simulink library "Simple_lib"  (R2018b)
settings: Solver=ode45  StartTime=0.0  StopTime=10.0  RelTol=1e-3  EnableMultiTasking=on
undefined symbols (not defined in the file or in its folder): Acceptance, beta, C, C_J, C_P, c_wall, dGain, DiscIntNeverNeededParam, Duplex, Electrical_lib, grab, h_fe, i, i3, K_T, Kman, KmanCE, mu_s, n_rev, R_arm, Simplex, systemTs, tau_0, TinIC, Ts, w_0, wallMass, Watch_lib
libraries: $bdroot x407, PlantUtilityBlockset_lib x30, peGeneralControl x22, simulink x11
(part 2 of 14)

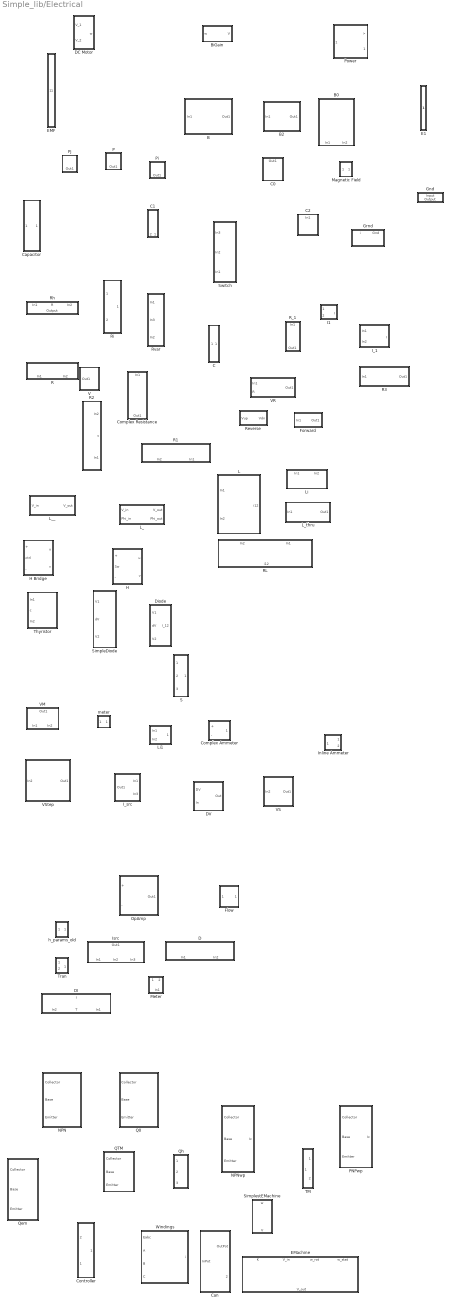
== system Simple_lib/Electrical ==
  B : Subsystem
      mask Display:
      | color('white')
      | plot([-1 1 1 -1 -1], [-1 -1 1 1 -1])
      | color('black')
      | 
      | plot([1.0 1.12 1.12 1.0], [0 .1 -.1 0])
      | plot([-1 -1], [-.4 .4])
      | plot([-.88 -.88], [-1 1])
      | plot([.88 .88], [-.4 .4])
      | plot([1 1], [-1 1])
      | 
      | plot([-.85 -.80], [0 0])
      | plot([-.7 -.6], [0 0])
      | plot([-.5 -.4], [0 0])
      | plot([-.3 -.2], [0 0])
      | plot([-.1 .0], [0 0])
      | plot([.1 .2], [0 0])
      | plot([.3 .4], [0 0])
      | plot([.5 .6], [0 0])
      | plot([.7 .8], [0 0])
  B0 : Subsystem
      mask Display:
      | color('white')
      | plot([-1 1 1 -1 -1], [-2 -2 2 2 -2])
      | color('black')
      | 
      | %plot( [0 .1 -.1 0],[1.0 1.12 1.12 1.0])
      | plot( [-.4 .4],[-.88 -.88])
      | plot([-1 1],[-1 -1])
      | plot([-.4 .4],[1 1])
      | plot([-1 1], [.88 .88])
      | 
      | plot([0 0],[-.85 -.80])
      | plot([0 0],[-.7 -.6])
      | plot([0 0],[-.5 -.4])
      | plot([0 0],[-.3 -.2])
      | plot([0 0],[-.1 .0])
      | plot([0 0],[.1 .2])
      | plot([0 0],[.3 .4])
      | plot([0 0],[.5 .6])
      | plot([0 0],[.7 .8])
  B2 : Subsystem
      mask Display:
      | plot([0 0], [-.4 .4])
      | plot([.06 .06], [-1 1])
      | plot([.94 .94], [-.4 .4])
      | 
      | plot([1 1], [-1 1])
      | plot([.06 .1], [0 0])
      | plot([.16 .2], [0 0])
      | plot([.26 .3], [0 0])
      | plot([.36 .4], [0 0])
      | plot([.46 .5], [0 0])
      | plot([.56 .6], [0 0])
      | plot([.66 .7], [0 0])
      | plot([.76 .8], [0 0])
      | plot([.86 .9], [0 0])
  BiGain : Subsystem  mask{k_level=-1, k_flow=-1}
      mask prompts: k_level "Potential Gain"; k_flow "Flow Gain"
      settings: AttributesFormatString="%<k_flow>   %<k_level>"
      mask Display:
      | patch( [0 1 0],[1 0 -1])
      | color('green')
      | plot( [0 -1 0],[1 0 -1])
  C : Subsystem  mask{C=100e-6}
      mask prompts: C "Capacitance"
      settings: AttributesFormatString=%<C>F
      mask Display:
      | %plot([1.0 1.8 1.8 1.0], [0 .1 -.1 0])
      | patch([-1 -1 -.7 -.7 -1], [-1 1 1 -1 -1])
      | patch([1 1 .7 .7 1], [-1 1 1 -1 -1])
  C0 : Subsystem
      mask Display:
      | plot(1-[0 0],[-1 1])
      | plot(1-[-0.4 -0.4],[-1 1])
      | plot(1-[0.6 0.6], [-0.6 0.6])
      | plot(1-[0.8 0.8],[-0.2 0.2])
      | 
      | plot(1-[-0.4 -1], [0 0])
      | plot(1-[0 0.6],[0 0])
  C1 : Subsystem  mask{C=1}
      mask prompts: C "Capacitance"
      mask Display:
      | color('white')
      | plot([-1 1 1 -1 -1], [-1 -1 1 1 -1])
      | color('black')
      | 
      | plot([-1 1], [0.5 0.5])
      | plot([-1 1], [-0.5 -0.5])
  C2 : Subsystem
      mask Display:
      | color('white')
      | plot([-1 1 1 -1 -1], [-1 -1 1 1 -1])
      | 
      | color('black')
      | %plot([1.0 1.18 1.18 1.0], [0 .15 -.15 0])
      | plot([0 0],[-1 1])
      | plot([-0.4 -0.4],[-1 1])
      | plot([0.6 0.6], [-0.6 0.6])
      | plot([0.8 0.8],[-0.2 0.2])
      | 
      | plot([-0.4 -1], [0 0])
      | plot([0 0.6],[0 0])
  Can : Subsystem  Tag=Electrical  AncestorBlock=Watch_lib/Acceptance  InitFcn=initCan
      mask Display:
      | %color('white')
      | %plot([0 3], [2 2])
      | %plot([0 3], [-2 -2])
      | %color('black')
      | 
      | plot([-1 -1 -.8 -.3 .3 .8 1 1], [1.5 -1.5 -1.8 -2 -2 -1.8 -1.5 1.5])
      | patch([-1 -.8 -.3 .3 .8 1 .8 .3 -.3 -.8 -1],[1.5 1.3 1.1 1.1 1.3 1.5 1.8 2 2 1.8 1.5])
  Capacitor : Subsystem  mask{C=.01}
      mask prompts: C "Capacitance"
      settings: AttributesFormatString=%<C>F
      mask Display:
      | %plot([1.0 1.8 1.8 1.0], [0 .1 -.1 0])
      | patch([-1 -1 -.7 -.7 -1], [-1 1 1 -1 -1])
      | patch([1 1 .7 .7 1], [-1 1 1 -1 -1])
  Complex Ammeter : Subsystem
      mask Display:
      | plot([-1 -.9 -.5 0 .5 .9 1  .9  .5  0 -.5 -.9 -1],      [ 0  .5 .9 1 .9 .5 0 -.5 -.9 -1 -.9 -.5  0]);
      | %plot([0 0], [0 -0.8])
      | %plot([0.2 0 -0.2], -[0.7 0.8 0.7])
      | port_label('input',1,'  +')
      | port_label('input',2,'  -')
      | disp('A')
  Complex Resistance : Subsystem  mask{R=0.01}
      mask prompts: R "Resistance"
      settings: AttributesFormatString=%<R> Ohm
      mask Display:
      | %color('black')
      | %plot([1.0 1.18 1.18 1.0], [0 .2 -.2 0])
      | plot([-8:8]/8, [0 1 0 -1 0 1 0 -1 0 1 0 -1 0 1 0 -1 0])
      | 
      | color('white')
      | plot([-1 1 1 -1 -1], [-1 -1 1 1 -1])
  Controller : Subsystem  InitFcn=initSimplex
      mask Display:
      | %color('white')
      | %plot([0 3], [2 2])
      | %plot([0 3], [-2 -2])
      | %color('black')
      | 
      | %plot([0 2 2 3], [1 1 0 0])
      | %plot([1 3 2 1 0 2], [0.6 0.6 0.4 0.6 0.4 0.4])
      | %patch([1 3 2],[0.6 0.6 0.4],[0,0,0])
      | %plot([0 1 1], [1 1 0.6])
      | %plot([1 1 0], [0.4 -1 -1])
      | 
      | plot( [0 0 0.15 .9 1 1 .9 0.15 0], [-.96 .96 1 .85 .8 -.8 -.85 -1 -.96])
      | patch( [.3 .4 .4 .3], [-.03 -.03 .03 .03])
      | patch( [.3 .4 .4 .3], [-.03 -.03 .03 .03]+.4)
      | patch( [.3 .4 .4 .3], [-.03 -.03 .03 .03]+.8)
      | patch( [.3 .4 .4 .3], [-.03 -.03 .03 .03]-.4)
      | patch( [.3 .4 .4 .3], [-.03 -.03 .03 .03]-.8)
      | patch( [.3 .4 .4 .3]+.4, [-.03 -.03 .03 .03]-.2)
      | patch( [.3 .4 .4 .3]+.4, [-.03 -.03 .03 .03]+.2)
      | patch( [.3 .4 .4 .3]+.4, [-.03 -.03 .03 .03]-.6)
      | patch( [.3 .4 .4 .3]+.4, [-.03 -.03 .03 .03]+.6)
  D : Subsystem
      mask Display:
      | plot( [ -1 0 0 ],[-1 -1 -0.3 ])
      | plot( [ 0 0 -1],[ 0.3 1 1])
      | plot( [ -1 1],-[1 1]*.3)
      | plot([-1 1 0 -1],[1 1 -1 1]*.3)
      | color('white')
      | plot([-1 1 1 -1 -1], [-1 -1 1 1 -1]*2)
      | %port_label('input', 1, '1')
  DC Motor : Subsystem  mask{k_flow=.1, J_mot=1e-4, R_arm=5, R_Fe=40}
      mask prompts: k_flow "Torque constant (Nm/A)"; J_mot "Intertia  (kgm^2)"; R_arm "Armature resistance (Ohm)"; R_Fe "R_Fe (Ohms)"
      mask Display:
      | %color('black')
      | %plot( [ -1 0  ],[-1 -1 ])
      | %plot( [ -1 0 ],[ 1 1])
      | 
      | plot([-1 -.9 -.5 0 .5 .9 1  .9  .5  0 -.5 -.9 -1],      [ 0  .5 .9 1 .9 .5 0 -.5 -.9 -1 -.9 -.5  0]);
      | %patch([0 1 1 0 0]-.5,[0 0 1 1 0]*.5-1.5,[0,0,1])
      | %patch([0 1 1 0 0]-.5,[0 0 1 1 0]*.5+1,[0,0,1])
      | color('blue')
      | plot([0 1 1 0 0]-.5,[0 0 1 1 0]*.5-1.5)
      | plot([0 1 1 0 0]-.5,[0 0 1 1 0]*.5+1)
      | %port_label('input', 1, '+')
      | %port_label('input', 2, '-')
      | %port_label('output', 1, 'V')
      | %color('white')
      | %plot([-1 1 1 -1 -1], [-1 -1 1 1 -1]*2)
  DI : Subsystem
      mask Display:
      | plot( [ -1 0 0 ],[-1 -1 -0.3 ])
      | plot( [ 0 0 -1],[ 0.3 1 1])
      | plot( [ -1 1],-[1 1]*.3)
      | plot([-1 1 0 -1],[1 1 -1 1]*.3)
      | color('white')
      | plot([-1 1 1 -1 -1], [-1 -1 1 1 -1]*2)
      | %port_label('input', 1, '1')
  DV : Subsystem
      mask Display:
      | port_label('input', 1, '-')
      | %port_label('input', 2, '-')
      | port_label('output', 1, '+')
      | 
      | plot([-1 0 1 0 -1],[0 0.7 0 -0.7 0])
  Diode : Subsystem
      mask Display:
      | plot( [ -1 0 0 ],[-1 -1 -0.3 ])
      | plot( [ 0 0 -1],[ 0.3 1 1])
      | plot( [ -1 1],-[1 1]*.3)
      | patch([-1 1 0 -1],[1 1 -1 1]*.3)
      | color('white')
      | plot([-1 1 1 -1 -1], [-1 -1 1 1 -1]*1.4)
      | %port_label('input', 1, '1')
  E1 : Subsystem
      mask Display:
      | plot([-1 -1], 0.5*[-1 1])
      | plot([1 1], [-1 1])
  EMF : Subsystem  mask{Vbatt=4}
      mask prompts: Vbatt "Voltage (V)"
      settings: AttributesFormatString=EMF: %<Vbatt> V
      mask Display:
      | %color('black')
      | plot([-1 -1], [-0.5 0.5])
      | plot([1 1], [-1 1.0])
      | %color('white')
      | %plot([-1 1 1 -1 -1], [-1 -1 1 1 -1])
  "EMachine " : Subsystem
  Flow : Subsystem
      mask Display:
      | plot( [-1 1 1 -1 -1], [-1 -1 1 1 -1] );
      | plot( 0.6*[-1 1 1 -1 -1], 0.3 + 0.5*[-1 -1 1 1 -1] );
  Forward : Subsystem  mask{deltaV=0}
      mask prompts: deltaV "Potential Drop (V)"
      mask Display:
      | patch( [1 1.05 1.05 1],[-1 -1 1 1])
      | patch( [1 0 0],[0 1 -1])
  Gnd : Subsystem
      mask Display:
      | color('cyan')
      | plot([-0.8 -0.8],[-1 1])
      | plot([-0.6 -0.6], [-0.6 0.6])
      | plot([-0.4 -0.4],[-0.2 0.2])
  Grnd : Subsystem
      mask Display:
      | %color('black')
      | %plot([1.0 1.18 1.18 1.0], [0 .15 -.15 0])
      | 
      | plot([-0.1 -0.1],[-1 1])
      | plot([-0.3 -0.3], [-0.6 0.6])
      | plot([-0.5 -0.5],[-0.2 0.2])
      | 
      | plot([-0.1 -0.5],[-1.5 -1.5])
      | 
      | %color('white')
      | %plot([-1 1 1 -1 -1], [-1 -1 1 1 -1])
  H : Subsystem
      mask Display: disp('H')
  H Bridge : Subsystem
      mask Display: disp('H')
  I1 : Subsystem
      mask Display:
      | color('cyan')
      | plot([-1 -.9 -.5 0 .5 .9 1  .9  .5  0 -.5 -.9 -1],...
      |   [ 0  .5 .9 1 .9 .5 0 -.5 -.9 -1 -.9 -.5  0]);
      | %plot([0 0], [0 -0.8])
      | %plot([0.2 0 -0.2], -[0.7 0.8 0.7])
      | port_label('input',1,' +')
      | %port_label('port_type', port_number, 'label', 'texmode', 'on')
      | port_label('input',2,' -')
      | disp(' A')
      | %text(0.2, 0.5, 'A', 'horizontalAlignment', 'center','texmode','on')
      | %color('white')
      | %plot( [-1.4 -1], [1,1])
  I_1 : Subsystem
  I_src : Subsystem
      mask Display:
      | %plot( [ -.5 0 0 ],[-1.3 -1.3 -0.7 ])
      | %plot( [ 0 0 -.5],[ 0.7 1.3 1.3])
      | plot( [ .2 0 -.2],[ -0.4 -.5 -.4])
      | plot( [ 0 0 ],[-1 1]*.5)
      | plot([-1 0 1 0 -1],[0 0.7 0 -0.7 0])
      | %port_label('input', 1, '+')
      | %port_label('output', 1, 'V')
      | %port_label('input', 3, '-')
      | %color('white')
      | %plot([-1 1 1 -1 -1], [-1 -1 1 1 -1]*2)
  Inline Ammeter : Subsystem
      mask Display:
      | %color('white')
      | %plot([-1 1 1 -1 -1], [-1 -1 1 1 -1])
      | %color('black')
      | %plot([1.0 1.18 1.18 1.0], [0 .2 -.2 0]+.4)
      | plot([-1 -.9 -.5 0 .5 .9 1  .9  .5  0 -.5 -.9 -1],      [ 0  .5 .9 1 .9 .5 0 -.5 -.9 -1 -.9 -.5  0]);
      | text(.4,-.4, 'A')
      | 
      | %color('white')
      | %plot([-1 1 1 -1 -1], [-1 -1 1 1 -1])
  Isrc : Subsystem
      mask Display:
      | plot( [ -.5 0 0 ],[-1.3 -1.3 -0.7 ])
      | plot( [ 0 0 -.5],[ 0.7 1.3 1.3])
      | plot( [ .2 0 -.2],[ -0.4 -.5 -.4])
      | plot( [ 0 0 ],[-1 1]*.5)
      | plot([-1 0 1 0 -1],[0 0.7 0 -0.7 0])
      | port_label('input', 1, '+')
      | port_label('output', 1, 'V')
      | port_label('input', 3, '-')
      | color('white')
      | plot([-1 1 1 -1 -1], [-1 -1 1 1 -1]*2)
  L : Subsystem  mask{L=200e-6}
      mask prompts: L "Inductance (H)"
      mask Display:
      | %color('black')
      | plot(   [    0     0.3827     0.7071     0.9239     1.0000     0.9239     0.7071     0.3827     0.0000    -0.3827    -0.7071    -0.9239    -1.0000    -0.9239    -0.7071    -0.3827    -0.0000     0.3827     0.7071     0.9239     1.0000     0.9239     0.7071     0.3827     0.0000    -0.3827    -0.7071    -0.9239    -1.0000    -0.9239    -0.7071    -0.3827    -0.0000     0.3827     0.7071     0.9239     1.0000     0.9239     0.7071     0.3827     0.0000    -0.3827    -0.7071    -0.9239    -1.0000    -0.9239    -0.7071    -0.3827    -0.0000     0.3827     0.7071     0.9239     1.0000     0.9239     0.7071     0.3827     0.0000    -0.3827    -0.7071    -0.9239    -1.0000    -0.9239    -0.7071    -0.3827    -0.0000],   -.5+[-0.0625    -0.0421    -0.0129     0.0230     0.0625     0.1020     0.1379     0.1671     0.1875     0.1984     0.2004     0.1958     0.1875     0.1792     0.1746     0.1766     0.1875     0.2079     0.2371     0.2730     0.3125     0.3520     0.3879     0.4171     0.4375     0.4484     0.4504     0.4458     0.4375     0.4292     0.4246     0.4266     0.4375     0.4579     0.4871     0.5230     0.5625     0.6020     0.6379     0.6671     0.6875     0.6984     0.7004     0.6958     0.6875     0.6792     0.6746     0.6766     0.6875     0.7079     0.7371     0.7730     0.8125     0.8520     0.8879     0.9171     0.9375     0.9484     0.9504     0.9458     0.9375     0.9292     0.9246     0.9266     0.9375])
      | color('white')
      | plot([-1 1 1 -1 -1], [-1 -1 1 1 -1])
  L_ : Subsystem  mask{L_turn=0.0001, N=200}
      mask prompts: L_turn "Inductance per turn"; N "N turns"
      settings: AttributesFormatString=%<L>H
      mask Display:
      | %color('white')
      | %plot([-1 1 1 -1 -1], [-1 -1 1 1 -1])
      | %color('black')
      | %plot([1.0 1.18 1.18 1.0], [0 .2 -.2 0])
      | plot(-1+2*[-0.0625
      |    -0.0421
      |    -0.0129
      |     0.0230
      |     0.0625
      |     0.1020
      |     0.1379
      |     0.1671
      |     0.1875
      |     0.1984
      |     0.2004
      |     0.1958
      |     0.1875
      |     0.1792
      |     0.1746
      |     0.1766
      |     0.1875
      |     0.2079
      |     0.2371
      |     0.2730
      |     0.3125
      |     0.3520
      |     0.3879
      |     0.4171
      |     0.4375
      |     0.4484
      |     0.4504
      |     0.4458
      |     0.4375
      |     0.4292
      |     0.4246
      |     0.4266
      |     0.4375
      |     0.4579
      |     0.4871
      |     0.5230
      |     0.5625
      |     0.6020
      |     0.6379
      |     0.6671
      |     0.6875
      |     0.6984
      |     0.7004
      |     0.6958
      |     0.6875
      |     0.6792
      |     0.6746
      |     0.6766
      |     0.6875
      |     0.7079
      |     0.7371
      |     0.7730
      |     0.8125
      |     0.8520
      |     0.8879
      |     0.9171
      |     0.9375
      |     0.9484
      |     0.9504
      |     0.9458
      |     0.9375
      |     0.9292
      |     0.9246
      |     0.9266
      |     0.9375], [    0
      |     0.3827
      |     0.7071
      |     0.9239
      |     1.0000
      |     0.9239
      |     0.7071
      |     0.3827
      |     0.0000
      |    -0.3827
      |    -0.7071
      |    -0.9239
      |    -1.0000
      |    -0.9239
      |    -0.7071
      |    -0.3827
      |    -0.0000
      |     0.3827
      |     0.7071
      |     0.9239
      |     1.0000
      |     0.9239
      |     0.7071
      |     0.3827
      |     0.0000
      |    -0.3827
      |    -0.7071
      |    -0.9239
      |    -1.0000
      |    -0.9239
      |    -0.7071
      |    -0.3827
      |    -0.0000
      |     0.3827
      |     0.7071
      |     0.9239
      |     1.0000
      |     0.9239
      |     0.7071
      |     0.3827
      |     0.0000
      |    -0.3827
      |    -0.7071
      |    -0.9239
      |    -1.0000
      |    -0.9239
      |    -0.7071
      |    -0.3827
      |    -0.0000
      |     0.3827
      |     0.7071
      |     0.9239
      |     1.0000
      |     0.9239
      |     0.7071
      |     0.3827
      |     0.0000
      |    -0.3827
      |    -0.7071
      |    -0.9239
      |    -1.0000
      |    -0.9239
      |    -0.7071
      |    -0.3827
      |    -0.0000])
  L__ : Subsystem  mask{L=1}
      mask prompts: L "Inductance"
      mask Display:
      | %color('white')
      | %plot([-1 1 1 -1 -1], [-1 -1 1 1 -1])
      | %color('black')
      | %plot([1.0 1.18 1.18 1.0], [0 .2 -.2 0])
      | plot(-1+2*[-0.0625
      |    -0.0421
      |    -0.0129
      |     0.0230
      |     0.0625
      |     0.1020
      |     0.1379
      |     0.1671
      |     0.1875
      |     0.1984
      |     0.2004
      |     0.1958
      |     0.1875
      |     0.1792
      |     0.1746
      |     0.1766
      |     0.1875
      |     0.2079
      |     0.2371
      |     0.2730
      |     0.3125
      |     0.3520
      |     0.3879
      |     0.4171
      |     0.4375
      |     0.4484
      |     0.4504
      |     0.4458
      |     0.4375
      |     0.4292
      |     0.4246
      |     0.4266
      |     0.4375
      |     0.4579
      |     0.4871
      |     0.5230
      |     0.5625
      |     0.6020
      |     0.6379
      |     0.6671
      |     0.6875
      |     0.6984
      |     0.7004
      |     0.6958
      |     0.6875
      |     0.6792
      |     0.6746
      |     0.6766
      |     0.6875
      |     0.7079
      |     0.7371
      |     0.7730
      |     0.8125
      |     0.8520
      |     0.8879
      |     0.9171
      |     0.9375
      |     0.9484
      |     0.9504
      |     0.9458
      |     0.9375
      |     0.9292
      |     0.9246
      |     0.9266
      |     0.9375], [    0
      |     0.3827
      |     0.7071
      |     0.9239
      |     1.0000
      |     0.9239
      |     0.7071
      |     0.3827
      |     0.0000
      |    -0.3827
      |    -0.7071
      |    -0.9239
      |    -1.0000
      |    -0.9239
      |    -0.7071
      |    -0.3827
      |    -0.0000
      |     0.3827
      |     0.7071
      |     0.9239
      |     1.0000
      |     0.9239
      |     0.7071
      |     0.3827
      |     0.0000
      |    -0.3827
      |    -0.7071
      |    -0.9239
      |    -1.0000
      |    -0.9239
      |    -0.7071
      |    -0.3827
      |    -0.0000
      |     0.3827
      |     0.7071
      |     0.9239
      |     1.0000
      |     0.9239
      |     0.7071
      |     0.3827
      |     0.0000
      |    -0.3827
      |    -0.7071
      |    -0.9239
      |    -1.0000
      |    -0.9239
      |    -0.7071
      |    -0.3827
      |    -0.0000
      |     0.3827
      |     0.7071
      |     0.9239
      |     1.0000
      |     0.9239
      |     0.7071
      |     0.3827
      |     0.0000
      |    -0.3827
      |    -0.7071
      |    -0.9239
      |    -1.0000
      |    -0.9239
      |    -0.7071
      |    -0.3827
      |    -0.0000])
  L_thru : Subsystem  mask{L=1}
      mask prompts: L "Inductance"
      mask Display:
      | color('white')
      | plot([-1 1 1 -1 -1], [-1 -1 1 1 -1])
      | color('black')
      | plot([1.0 1.18 1.18 1.0], [0 .2 -.2 0])
      | plot(-1+2*[-0.0625
      |    -0.0421
      |    -0.0129
      |     0.0230
      |     0.0625
      |     0.1020
      |     0.1379
      |     0.1671
      |     0.1875
      |     0.1984
      |     0.2004
      |     0.1958
      |     0.1875
      |     0.1792
      |     0.1746
      |     0.1766
      |     0.1875
      |     0.2079
      |     0.2371
      |     0.2730
      |     0.3125
      |     0.3520
      |     0.3879
      |     0.4171
      |     0.4375
      |     0.4484
      |     0.4504
      |     0.4458
      |     0.4375
      |     0.4292
      |     0.4246
      |     0.4266
      |     0.4375
      |     0.4579
      |     0.4871
      |     0.5230
      |     0.5625
      |     0.6020
      |     0.6379
      |     0.6671
      |     0.6875
      |     0.6984
      |     0.7004
      |     0.6958
      |     0.6875
      |     0.6792
      |     0.6746
      |     0.6766
      |     0.6875
      |     0.7079
      |     0.7371
      |     0.7730
      |     0.8125
      |     0.8520
      |     0.8879
      |     0.9171
      |     0.9375
      |     0.9484
      |     0.9504
      |     0.9458
      |     0.9375
      |     0.9292
      |     0.9246
      |     0.9266
      |     0.9375], [    0
      |     0.3827
      |     0.7071
      |     0.9239
      |     1.0000
      |     0.9239
      |     0.7071
      |     0.3827
      |     0.0000
      |    -0.3827
      |    -0.7071
      |    -0.9239
      |    -1.0000
      |    -0.9239
      |    -0.7071
      |    -0.3827
      |    -0.0000
      |     0.3827
      |     0.7071
      |     0.9239
      |     1.0000
      |     0.9239
      |     0.7071
      |     0.3827
      |     0.0000
      |    -0.3827
      |    -0.7071
      |    -0.9239
      |    -1.0000
      |    -0.9239
      |    -0.7071
      |    -0.3827
      |    -0.0000
      |     0.3827
      |     0.7071
      |     0.9239
      |     1.0000
      |     0.9239
      |     0.7071
      |     0.3827
      |     0.0000
      |    -0.3827
      |    -0.7071
      |    -0.9239
      |    -1.0000
      |    -0.9239
      |    -0.7071
      |    -0.3827
      |    -0.0000
      |     0.3827
      |     0.7071
      |     0.9239
      |     1.0000
      |     0.9239
      |     0.7071
      |     0.3827
      |     0.0000
      |    -0.3827
      |    -0.7071
      |    -0.9239
      |    -1.0000
      |    -0.9239
      |    -0.7071
      |    -0.3827
      |    -0.0000])
  Li : Subsystem  mask{L=1e-3}
      mask prompts: L "Inductance (H)"
      mask Display:
      | %color('black')
      | plot(   [    0     0.3827     0.7071     0.9239     1.0000     0.9239     0.7071     0.3827     0.0000    -0.3827    -0.7071    -0.9239    -1.0000    -0.9239    -0.7071    -0.3827    -0.0000     0.3827     0.7071     0.9239     1.0000     0.9239     0.7071     0.3827     0.0000    -0.3827    -0.7071    -0.9239    -1.0000    -0.9239    -0.7071    -0.3827    -0.0000     0.3827     0.7071     0.9239     1.0000     0.9239     0.7071     0.3827     0.0000    -0.3827    -0.7071    -0.9239    -1.0000    -0.9239    -0.7071    -0.3827    -0.0000     0.3827     0.7071     0.9239     1.0000     0.9239     0.7071     0.3827     0.0000    -0.3827    -0.7071    -0.9239    -1.0000    -0.9239    -0.7071    -0.3827    -0.0000],   -.5+[-0.0625    -0.0421    -0.0129     0.0230     0.0625     0.1020     0.1379     0.1671     0.1875     0.1984     0.2004     0.1958     0.1875     0.1792     0.1746     0.1766     0.1875     0.2079     0.2371     0.2730     0.3125     0.3520     0.3879     0.4171     0.4375     0.4484     0.4504     0.4458     0.4375     0.4292     0.4246     0.4266     0.4375     0.4579     0.4871     0.5230     0.5625     0.6020     0.6379     0.6671     0.6875     0.6984     0.7004     0.6958     0.6875     0.6792     0.6746     0.6766     0.6875     0.7079     0.7371     0.7730     0.8125     0.8520     0.8879     0.9171     0.9375     0.9484     0.9504     0.9458     0.9375     0.9292     0.9246     0.9266     0.9375])
      | color('white')
      | plot([-1 1], [-1 -1])
      | plot([-1 1], [1 1])
  Li1 : Subsystem
      mask Display:
      | plot([-1 -.9 -.5 0 .5 .9 1  .9  .5  0 -.5 -.9 -1],      [ 0  .5 .9 1 .9 .5 0 -.5 -.9 -1 -.9 -.5  0]);
      | plot([0 0], [0 -0.8])
      | plot([0.2 0 -0.2], -[0.7 0.8 0.7])
  Magnetic Field : Subsystem  mask{k_lev=0, k_flo=0}
      mask prompts: k_lev "Level Gain"; k_flo "Flow Gain"
      mask Display:
      | %patch( [1 1.05 1.05 1],[-1 -1 1 1])
      | patch( [1 0 0],[0 1 -1])
      | plot( [0 1 1],[1 2 0])
  Meter : Subsystem
      mask Display:
      | %color('white')
      | %plot([-1 1 1 -1 -1], [-1 -1 1 1 -1])
      | %color('black')
      | plot([1.0 1.18 1.18 1.0], [0 .2 -.2 0]+.4)
      | plot([-1 -.9 -.5 0 .5 .9 1  .9  .5  0 -.5 -.9 -1],      [ 0  .5 .9 1 .9 .5 0 -.5 -.9 -1 -.9 -.5  0]);
      | text(.4,-.4, 'A')
      | 
      | %color('white')
      | %plot([-1 1 1 -1 -1], [-1 -1 1 1 -1])
  NPN : Subsystem  mask{h_fe=beta, Kman=Kman}
      mask prompts: h_fe "h_fe (-)"
      mask Display:
      | patch([0 0 0.1 0.1],[-1 1 1 -1])
      | 
      | plot([0 1],[0.25 1])
      | plot([0 1],[-0.25 -1])
      | 
      | patch([.8 1 1],[-1 -1 -0.8])
  NPNwp : Subsystem
      mask Display:
      | patch([0 0 0.1 0.1],[-1 1 1 -1])
      | 
      | plot([0 1],[0.25 1])
      | plot([0 1],[-0.25 -1])
      | 
      | patch([.8 1 1],[-1 -1 -0.8])
  OpAmp : Subsystem  mask{K_op=1000}
      mask prompts: K_op "K_op (Hz)"
      mask Display:
      | %patch( [1 1.05 1.05 1],[-1 -1 1 1])
      | plot( [1 0 0 1],[0 1 -1 0])
      | port_label('input', 1, '+')
      | port_label('input', 2, '-')
  P : Subsystem
      mask Display: disp(get(gcbh,'Name'))
  PNPwp : Subsystem
      mask Display:
      | patch([0 0 0.1 0.1],[-1 1 1 -1])
      | 
      | plot([0 1],[0.25 1])
      | plot([0 1],[-0.25 -1])
      | 
      | patch([.1 .35 .2],[-0.25 -0.35 -0.5])
  Pi : Subsystem
      mask Display: disp(get(gcbh,'Name'))
  Pj : Subsystem
      mask Display: disp(get(gcbh,'Name'))
  Power : Subsystem
      mask Display:
      | plot([-1 -.9 -.5 0 .5 .9 1  .9  .5  0 -.5 -.9 -1],      [ 0  .5 .9 1 .9 .5 0 -.5 -.9 -1 -.9 -.5  0]);
      | disp('P')
  Q0 : Subsystem  mask{h_fe=beta, Kman=Kman}
      mask prompts: h_fe "h_fe (-)"
      mask Display:
      | patch([0 0 0.1 0.1],[-1 1 1 -1])
      | 
      | plot([0 1],[0.25 1])
      | plot([0 1],[-0.25 -1])
      | 
      | patch([.8 1 1],[-1 -1 -0.8])
  QTM : Subsystem  mask{h_fe=100, Kman=100}
      mask prompts: h_fe "h_fe (-)"
      mask Display:
      | patch([0 0 0.1 0.1],[-1 1 1 -1])
      | 
      | plot([0 1],[0.25 1])
      | plot([0 1],[-0.25 -1])
      | 
      | patch([.8 1 1],[-1 -1 -0.8])
  Qem : Subsystem
      mask Display:
      | patch([0 0 0.1 0.1],[-1 1 1 -1])
      | 
      | plot([0 1],[0.25 1])
      | plot([0 1],[-0.25 -1])
      | 
      | patch([.8 1 1],[-1 -1 -0.8])
  Qh : Subsystem  mask{h_re=1e-3, h_fe=100, h_ie=1e3, h_oe=1e6}
      mask prompts: h_re "h_re (-)"; h_fe "h_fe (-)"; h_ie "h_ie (ohms)"; h_oe "h_oe (ohms)"
      mask Display:
      | patch([0 0 0.1 0.1],[-1 1 1 -1])
      | 
      | plot([0 1],[0.25 1])
      | plot([0 1],[-0.25 -1])
      | 
      | patch([.8 1 1],[-1 -1 -0.8])
  R : Subsystem  mask{R=1}
      mask prompts: R "Resistance (Ohms)"
      settings: AttributesFormatString=%<R> Ohms
      mask Display:
      | %color('black')
      | plot( [ -1 1 -1 1 -1 1 -1],[-3:3]/6)
      | 
      | color('white')
      | plot([-1 1 1 -1 -1], [-1 -1 1 1 -1])
  R1 : Subsystem  mask{R=.5}
      mask prompts: R "Resistance"
      mask Display:
      | %color('black')
      | plot( [ -1 1 -1 1 -1 1 -1],[-3:3]/6)
      | 
      | color('white')
      | plot([-1 1 1 -1 -1], [-1 -1 1 1 -1])
  R2 : Subsystem  AncestorBlock=PlantUtilityBlockset_lib/Electrical/R1
      mask Display:
      | color('white')
      | plot([-1 1 1 -1 -1], [-1 -1 1 1 -1])
      | color('black')
      | plot( [ -1 0 1 0 -1 0 1 0 -1 0 1 0 -1],[-6:6]/12)
  R3 : Subsystem  mask{R=100}
      mask prompts: R "Resistance (Ohm)"
      settings: AttributesFormatString=%<R> Ohm
  RL : Subsystem  mask{R=100, L=.1}
      mask prompts: R "Resistance (Ohms)"; L "Inductance (H)"
      settings: AttributesFormatString=%<R> Ohms
      mask Display:
      | %color('black')
      | plot(   .4*[    0     0.3827     0.7071     0.9239     1.0000     0.9239     0.7071     0.3827     0.0000    -0.3827    -0.7071    -0.9239    -1.0000    -0.9239    -0.7071    -0.3827    -0.0000     0.3827     0.7071     0.9239     1.0000     0.9239     0.7071     0.3827     0.0000    -0.3827    -0.7071    -0.9239    -1.0000    -0.9239    -0.7071    -0.3827    -0.0000     0.3827     0.7071     0.9239     1.0000     0.9239     0.7071     0.3827     0.0000    -0.3827    -0.7071    -0.9239    -1.0000    -0.9239    -0.7071    -0.3827    -0.0000     0.3827     0.7071     0.9239     1.0000     0.9239     0.7071     0.3827     0.0000    -0.3827    -0.7071    -0.9239    -1.0000    -0.9239    -0.7071    -0.3827    -0.0000],   -.5+[-0.0625    -0.0421    -0.0129     0.0230     0.0625     0.1020     0.1379     0.1671     0.1875     0.1984     0.2004     0.1958     0.1875     0.1792     0.1746     0.1766     0.1875     0.2079     0.2371     0.2730     0.3125     0.3520     0.3879     0.4171     0.4375     0.4484     0.4504     0.4458     0.4375     0.4292     0.4246     0.4266     0.4375     0.4579     0.4871     0.5230     0.5625     0.6020     0.6379     0.6671     0.6875     0.6984     0.7004     0.6958     0.6875     0.6792     0.6746     0.6766     0.6875     0.7079     0.7371     0.7730     0.8125     0.8520     0.8879     0.9171     0.9375     0.9484     0.9504     0.9458     0.9375     0.9292     0.9246     0.9266     0.9375])
      | plot( [ -.4 .6 -.8 1 ],-.5+[-3:0]/6)
      | plot( [ -.4 .6 -.8 1 ],.5+[0:3]/6)
      | color('white')
      | plot([-1 1 1 -1 -1], [-1 -1 1 1 -1])
  R_1 : Subsystem  mask{R=1e3}
      mask prompts: R "Resistance"
      settings: AttributesFormatString=%<R> Ohm
      mask Display:
      | %color('black')
      | %plot([1.0 1.18 1.18 1.0], [0 .2 -.2 0])
      | plot([-8:8]/8, [0 1 0 -1 0 1 0 -1 0 1 0 -1 0 1 0 -1 0])
      | 
      | color('white')
      | plot([-1 1 1 -1 -1], [-1 -1 1 1 -1])
  Reverse : Subsystem  mask{deltaV=0}
      mask prompts: deltaV "Potential Drop (V)"
      mask Display:
      | patch( [0 -0.05 -0.05 0],[-1 -1 1 1])
      | patch( [0 1 1],[0 1 -1])
  Rh : Subsystem
      mask Display:
      | %plot( [ -1 1 -1 1 -1 1 -1],[-3:3]/6)
      | %plot( [ .2 0 -.2],[ -0.4 -.5 -.4])
      | plot( [ 0 1 1 -1 -1 0 ],[-2 -1.9 1 1 -1.9 -2])
      | 
      | color('white')
      | plot([-1 1], [1.1 1.1])
      | %color('red')
      | %plot([-1 1], -[2 2])
  Ri : Subsystem  mask{R=1}
      mask prompts: R "Resistance (Ohms)"
      settings: AttributesFormatString=%<R> Ohms
      mask Display:
      | %plot( [ -1 1 -1 1 -1 1 -1],[-3:3]/6)
      | %plot( [ .2 0 -.2],[ -0.4 -.5 -.4])
      | plot( [ 0 1 1 -1 -1 0 ],[-2 -1 1 1 -1 -2])
      | 
      | color('white')
      | plot([-1 1], [2 2])
      | %color('red')
      | %plot([-1 1], -[2 2])
  Rvar : Subsystem
      mask Display:
      | %plot( [ -1 1 -1 1 -1 1 -1],[-3:3]/6)
      | %plot( [ .2 0 -.2],[ -0.4 -.5 -.4])
      | plot( [ 0 1 1 -1 -1 0 ],[-2 -1.33 1.33 1.33 -1.33 -2])
      | 
      | color('white')
      | plot([-1 1], [2 2])
      | %color('red')
      | %plot([-1 1], -[2 2])
  S : Subsystem
      mask Display:
      | %plot([-1 -.9 -.5 0 .5 .9 1  .9  .5  0 -.5 -.9 -1],      [ 0  .5 .9 1 .9 .5 0 -.5 -.9 -1 -.9 -.5  0]);
      | %plot([0 0], [0 -0.8])
      | %plot([0.2 0 -0.2], -[0.7 0.8 0.7])
      | 
      | %color('black')
      | plot( [ 0 0 ], [ 1 .3 ]*2/3 )
      | plot( [ 0 0 ],-[ 1 .3 ]*2/3 )
      | plot( [ 1 1 ],[ -.3 .3 ]*2/3 )
      | patch([0.2 0 -0.2]+1, -[0.0 0.1 0.0]-.2)
      | 
      | color('white')
      | %plot([-1 .1 .1 -1 -1], [-1 -1 1 1 -1])
  SimpleDiode : Subsystem  mask{K_diode=KmanCE}
      mask prompts: K_diode "K_diode (s/Ohm)"
      mask Display:
      | plot( [ -1 0 0 ],[-1 -1 -0.3 ])
      | plot( [ 0 0 -1],[ 0.3 1 1])
      | plot( [ -1 1],-[1 1]*.3)
      | patch([-1 1 0 -1],[1 1 -1 1]*.3)
      | color('white')
      | plot([-1 1 1 -1 -1], [-1 -1 1 1 -1]*1.4)
      | %port_label('input', 1, '1')
  SimplestEMachine : Subsystem
  Switch : Subsystem
      settings: AttributesFormatString=%<R> Ohms
      mask Display:
      | %color('black')
      | plot( [ -1 0 0 ], [ 1 1 .3 ]*2/3 )
      | plot( [ -1 0 0 ],-[ 1 1 .3 ]*2/3 )
      | plot( [ -1 -1 ]/2,[ -.3 .3 ]*2/3 )
      | 
      | color('white')
      | plot([-1 1 1 -1 -1], [-1 -1 1 1 -1])
  TM : Subsystem
      mask Display:
      | patch([0 0 0.1 0.1],[-1 1 1 -1])
      | 
      | plot([0 1],[0.25 1])
      | plot([0 1],[-0.25 -1])
      | 
      | patch([.8 1 1],[-1 -1 -0.8])
      | color white
      | plot([0 1],2*[1  1])
      | plot([0 1],-2*[1  1])
  Thyristor : Subsystem  AncestorBlock=PlantUtilityBlockset_lib/Electrical/R1
      mask Display:
      | %color('black')
      | %plot( [ -1 0 1 0 -1 0 1 0 -1 0 1 0 -1],[-6:6]/12)
      | plot( [0 -1 1 0 1 -1 -.6 -1],-[.0 -.66 -.66 .0 .0 .0 .0 .66])
      | 
      | color('white')
      | plot([-1 1 1 -1 -1], [-1 -1 1 1 -1])
  Tran : Subsystem
      mask Display:
      | %patch( [1 1.05 1.05 1],[-1 -1 1 1])
      | patch( [1 0 0],[0 1 -1])
      | plot( [0 1 1],[1 2 0])
  V : Subsystem  mask{C=1}
      mask prompts: C "Capacitance"
      mask Display: disp(get(gcbh,'Name'))
  VM : Subsystem
      mask Display:
      | color('white')
      | plot([-1 1 1 -1 -1], [-1 -1 1 1 -1]*2)
      | color('black')
      | plot( [ -1 0  ],[-1 -1 ])
      | plot( [ -1 0 ],[ 1 1])
      | 
      | plot([-1 -.9 -.5 0 .5 .9 1  .9  .5  0 -.5 -.9 -1],      [ 0  .5 .9 1 .9 .5 0 -.5 -.9 -1 -.9 -.5  0]);
      | port_label('input', 1, '+')
      | port_label('input', 2, '-')
      | port_label('output', 1, 'V')
  VR : Subsystem
      mask Display:
      | %color('black')
      | %plot([1.0 1.18 1.18 1.0], [0 .2 -.2 0])
      | plot([-8:8]/8, [0 1 0 -1 0 1 0 -1 0 1 0 -1 0 1 0 -1 0])
      | plot([-1 1], [-.75 .75] )
      | patch([0.9 1 .95],[.75 .75 .5])
      | color('white')
      | %plot([-1 1 1 -1 -1], [-1 -1 1 1 -1])
  VS : Subsystem
      mask Display:
      | %color('white')
      | %plot([-1 1 1 -1 -1], [-1 -1 1 1 -1])
      | %color('black')
      | plot([1.0 1.18 1.18 1.0], [0 .2 -.2 0])
      | 
      | %color('white')
      | %plot([-1 1 1 -1 -1], [-1 -1 1 1 -1]*2)
      | %color('black')
      | %plot( [ -.5 0 0 ],[-1.3 -1.3 -0.7 ])
      | %plot( [ 0 0 -.5],[ 0.7 1.3 1.3])
      | %plot( [ .2 0 -.2],[ -0.4 -.5 -.4])
      | %plot( [ 0 0 ],[-1 1]*.5)
      | plot([-1 0 1 0 -1],[0 0.7 0 -0.7 0])
      | %port_label('input', 1, '+')
      | %port_label('output', 1, 'V')
      | %port_label('input', 3, '-')
  VStep : Subsystem  AncestorBlock=PlantUtilityBlockset_lib/Electrical/VS  mask{R=1}
      mask prompts: R "Resistance"
      mask Display:
      | color('white')
      | plot([-1 1 1 -1 -1], [-1 -1 1 1 -1])
      | color('black')
      | plot([1.0 1.18 1.18 1.0], [0 .2 -.2 0])
      | 
      | color('white')
      | plot([-1 1 1 -1 -1], [-1 -1 1 1 -1]*2)
      | color('black')
      | plot( [ -.5 0 0 ],[-1.3 -1.3 -0.7 ])
      | plot( [ 0 0 -.5],[ 0.7 1.3 1.3])
      | plot( [ .2 0 -.2],[ -0.4 -.5 -.4])
      | plot( [ 0 0 ],[-1 1]*.5)
      | plot([-1 0 1 0 -1],[0 0.7 0 -0.7 0])
      | port_label('input', 1, '+')
      | port_label('output', 1, 'V')
      | port_label('input', 3, '-')
  Windings : Subsystem
  h_params_old : Subsystem
      mask Display:
      | %patch( [1 1.05 1.05 1],[-1 -1 1 1])
      | patch( [1 0 0],[0 1 -1])
      | plot( [0 1 1],[1 2 0])
  meter : Subsystem
      mask Display: plot([-1 -.9 -.5 0 .5 .9 1  .9  .5  0 -.5 -.9 -1],      [ 0  .5 .9 1 .9 .5 0 -.5 -.9 -1 -.9 -.5  0]);
